simulink model "main_simulink"  (R2022a)
settings: Solver=VariableStepAuto  StartTime=0.0  StopTime=8  RelTol=1e-3
values from neighbouring files (symbols this model uses):
  A = 24    [main.m]
  a = 18    [main.m]
  b = 8    [main.m]
libraries: slpidlib x2, simulink_extras x2
settings Model: Creator=240818  LastModifiedBy=punk
settings DebuggingCC: UnconnectedInputMsg=warning  UnconnectedOutputMsg=warning  UnconnectedLineMsg=warning
settings RTWCC: DLArmComputeVersion=19.05

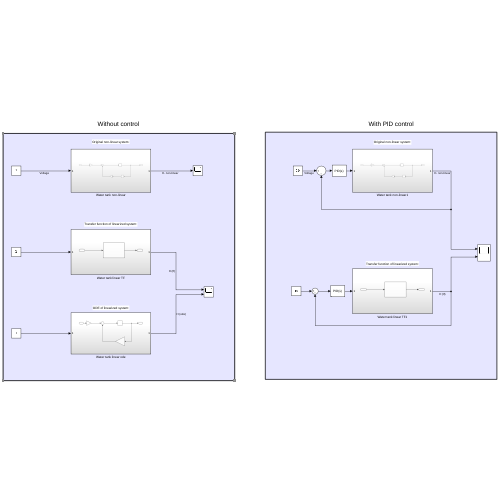
[thumbnail: Simulink's stored preview of the top-level diagram]
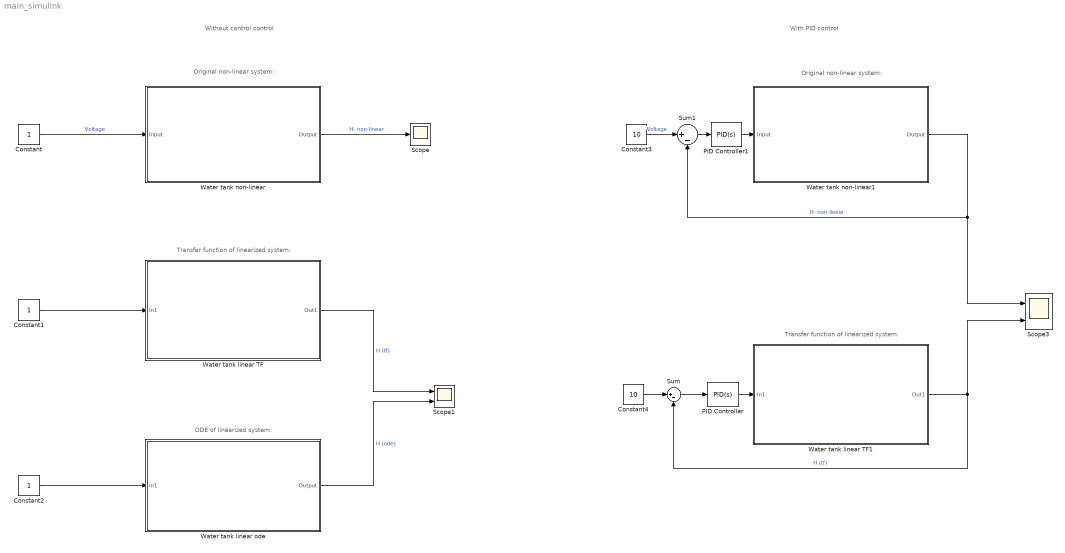
== system main_simulink ==
  note: With PID control
  note: ODE of linearized system:
  note: Transfer function of linearized system:
  note: Original non-linear system:
  note: Transfer function of linearized system:
  note: Original non-linear system:
  note: Without control control
  Constant : Constant
  Constant1 : Constant
  Constant2 : Constant
  Constant3 : Constant  Value=10
  Constant4 : Constant  Value=10
  PID Controller : slpidlib/PID Controller  Controller=PID  Form=Parallel  TimeDomain=Continuous-time  UseExternalTs=off  SampleTime=-1  IntegratorMethod=Forward Euler  FilterMethod=Forward Euler  ControllerParametersSource=internal  P=15  I=5  UseKiTs=off  D=1  N=0  UseFilter=on  TunerSelectOption=Transfer Function Based (PID Tuner App)  InitialConditionSource=internal  InitialConditionForIntegrator=0  InitialConditionForFilter=0  DifferentiatorICPrevScaledInput=0  ExternalReset=none  TrackingMode=off  Kt=1  LimitOutput=off  SatLimitsSource=internal  UpperSaturationLimit=inf  LowerSaturationLimit=-inf  LinearizeAsGain=on  AntiWindupMode=none  Kb=1  POutMin=[]  POutMax=[]  IOutMin=[]  IOutMax=[]  DOutMin=[]  DOutMax=[]  NOutMin=[]  NOutMax=[]  SumOutMin=[]  SumOutMax=[]  SaturationOutMin=[]  SaturationOutMax=[]  PParamMin=[]  PParamMax=[]  IParamMin=[]  IParamMax=[]  DParamMin=[]  DParamMax=[]  NParamMin=[]  NParamMax=[]  KbParamMin=[]  KbParamMax=[]  KtParamMin=[]  KtParamMax=[]  KbOutMin=[]  KbOutMax=[]  KtOutMin=[]  KtOutMax=[]  IntegratorOutMin=[]  IntegratorOutMax=[]  FilterOutMin=[]  FilterOutMax=[]  SumI1OutMin=[]  SumI1OutMax=[]  SumI2OutMin=[]  SumI2OutMax=[]  SumI3OutMin=[]  SumI3OutMax=[]  SumI4OutMin=[]  SumI4OutMax=[]  SumDOutMin=[]  SumDOutMax=[]  DifferentiatorOutMin=[]  DifferentiatorOutMax=[]  FilterDiffOutCoefMin=[]  FilterDiffOutCoefMax=[]  ReciprocalOutMin=[]  ReciprocalOutMax=[]  SumDenOutMin=[]  SumDenOutMax=[]  SumNumOutMin=[]  SumNumOutMax=[]  DivideOutMin=[]  DivideOutMax=[]  UdiffTsProdOutMin=[]  UdiffTsProdOutMax=[]  NTsProdOutMin=[]  NTsProdOutMax=[]  UintegralTsProdOutMin=[]  UintegralTsProdOutMax=[]  UngainTsProdOutMin=[]  UngainTsProdOutMax=[]  ClampingZeroOutDataTypeStr=Inherit: Inherit via back propagation  ClampingZeroOutMin=[]  ClampingZeroOutMax=[]  FilterDenConstantOutDataTypeStr=Inherit: Inherit via back propagation  FilterDenConstantOutMin=[]  FilterDenConstantOutMax=[]  PCopyOutDataTypeStr=Inherit: Inherit via back propagation  PCopyOutMin=[]  PCopyOutMax=[]  NCopyOutDataTypeStr=Inherit: Inherit via back propagation  NCopyOutMin=[]  NCopyOutMax=[]  IntegratorContinuousStateAttributes=''  IntegratorStateMustResolveToSignalObject=off  IntegratorRTWStateStorageClass=Auto  FilterContinuousStateAttributes=''  FilterStateMustResolveToSignalObject=off  FilterRTWStateStorageClass=Auto  ParallelPVariant=InternalParameters  IdealPVariant=Disabled  IVariant=InternalParameters  DVariant=InternalParameters  IntegratorVariant=Continuous  SatVariant=Disabled  AWVariant=Passthrough  PCopyVariant=Disabled  TRVariant=Disabled  FdbkBlocksVariant=Forward  IdealPFdbkVariant=Disabled  SatFdbkVariant=Disabled  DerivativeFilterVariant=ContFilter  NVariant=InternalParameters  NCopyVariant=Disabled  FilterICVariant=InternalICsFilter  IntegratorICVariant=InternalICs  ExternalResetVariant=Disabled  TRSumVariant=Passthrough  SumFdbkVariant=Disabled  SumVariant=Sum_PID  TsampFilterVariant=InternalTs  TsampNgainVariant=Passthrough  TsampIntegralVariant=Passthrough  ExternalSaturationOutDataTypeStr=Inherit: Same as second input  aMode=0
  PID Controller1 : slpidlib/PID Controller  Controller=PID  Form=Parallel  TimeDomain=Continuous-time  UseExternalTs=off  SampleTime=-1  IntegratorMethod=Forward Euler  FilterMethod=Forward Euler  ControllerParametersSource=internal  P=15  I=5  UseKiTs=off  D=1  N=0  UseFilter=on  TunerSelectOption=Transfer Function Based (PID Tuner App)  InitialConditionSource=internal  InitialConditionForIntegrator=0  InitialConditionForFilter=0  DifferentiatorICPrevScaledInput=0  ExternalReset=none  TrackingMode=off  Kt=1  LimitOutput=off  SatLimitsSource=internal  UpperSaturationLimit=inf  LowerSaturationLimit=-inf  LinearizeAsGain=on  AntiWindupMode=none  Kb=1  POutMin=[]  POutMax=[]  IOutMin=[]  IOutMax=[]  DOutMin=[]  DOutMax=[]  NOutMin=[]  NOutMax=[]  SumOutMin=[]  SumOutMax=[]  SaturationOutMin=[]  SaturationOutMax=[]  PParamMin=[]  PParamMax=[]  IParamMin=[]  IParamMax=[]  DParamMin=[]  DParamMax=[]  NParamMin=[]  NParamMax=[]  KbParamMin=[]  KbParamMax=[]  KtParamMin=[]  KtParamMax=[]  KbOutMin=[]  KbOutMax=[]  KtOutMin=[]  KtOutMax=[]  IntegratorOutMin=[]  IntegratorOutMax=[]  FilterOutMin=[]  FilterOutMax=[]  SumI1OutMin=[]  SumI1OutMax=[]  SumI2OutMin=[]  SumI2OutMax=[]  SumI3OutMin=[]  SumI3OutMax=[]  SumI4OutMin=[]  SumI4OutMax=[]  SumDOutMin=[]  SumDOutMax=[]  DifferentiatorOutMin=[]  DifferentiatorOutMax=[]  FilterDiffOutCoefMin=[]  FilterDiffOutCoefMax=[]  ReciprocalOutMin=[]  ReciprocalOutMax=[]  SumDenOutMin=[]  SumDenOutMax=[]  SumNumOutMin=[]  SumNumOutMax=[]  DivideOutMin=[]  DivideOutMax=[]  UdiffTsProdOutMin=[]  UdiffTsProdOutMax=[]  NTsProdOutMin=[]  NTsProdOutMax=[]  UintegralTsProdOutMin=[]  UintegralTsProdOutMax=[]  UngainTsProdOutMin=[]  UngainTsProdOutMax=[]  ClampingZeroOutDataTypeStr=Inherit: Inherit via back propagation  ClampingZeroOutMin=[]  ClampingZeroOutMax=[]  FilterDenConstantOutDataTypeStr=Inherit: Inherit via back propagation  FilterDenConstantOutMin=[]  FilterDenConstantOutMax=[]  PCopyOutDataTypeStr=Inherit: Inherit via back propagation  PCopyOutMin=[]  PCopyOutMax=[]  NCopyOutDataTypeStr=Inherit: Inherit via back propagation  NCopyOutMin=[]  NCopyOutMax=[]  IntegratorContinuousStateAttributes=''  IntegratorStateMustResolveToSignalObject=off  IntegratorRTWStateStorageClass=Auto  FilterContinuousStateAttributes=''  FilterStateMustResolveToSignalObject=off  FilterRTWStateStorageClass=Auto  ParallelPVariant=InternalParameters  IdealPVariant=Disabled  IVariant=InternalParameters  DVariant=InternalParameters  IntegratorVariant=Continuous  SatVariant=Disabled  AWVariant=Passthrough  PCopyVariant=Disabled  TRVariant=Disabled  FdbkBlocksVariant=Forward  IdealPFdbkVariant=Disabled  SatFdbkVariant=Disabled  DerivativeFilterVariant=ContFilter  NVariant=InternalParameters  NCopyVariant=Disabled  FilterICVariant=InternalICsFilter  IntegratorICVariant=InternalICs  ExternalResetVariant=Disabled  TRSumVariant=Passthrough  SumFdbkVariant=Disabled  SumVariant=Sum_PID  TsampFilterVariant=InternalTs  TsampNgainVariant=Passthrough  TsampIntegralVariant=Passthrough  ExternalSaturationOutDataTypeStr=Inherit: Same as second input  aMode=0
  Scope : Scope
  Scope1 : Scope  NumInputPorts=2
  Scope3 : Scope  NumInputPorts=2
  Sum : Sum  Inputs=|+-
  Sum1 : Sum  Inputs=|+-
  Water tank linear TF : Subsystem
  Water tank linear TF1 : Subsystem
  Water tank linear ode : Subsystem
  Water tank non-linear : Subsystem
  Water tank non-linear1 : Subsystem
  wires:
  Constant/1 -> Water tank non-linear/1(Input)  "Voltage"
  Water tank non-linear/1(Output) -> Scope/1  "H- non-linear"
  Constant1/1 -> Water tank linear TF/1(In1)
  Water tank linear TF/1(Out1) -> Scope1/1  "H (tf)"
  Constant2/1 -> Water tank linear ode/1(In1)
  Water tank linear ode/1(Output) -> Scope1/2  "H (ode)"
  Constant3/1 -> Sum1/1  "Voltage"
  Water tank linear TF1/1(Out1) -> Sum/2, Scope3/2  "H (tf)"
  PID Controller/1 -> Water tank linear TF1/1(In1)
  Sum/1 -> PID Controller/1
  Constant4/1 -> Sum/1
  PID Controller1/1 -> Water tank non-linear1/1(Input)
  Sum1/1 -> PID Controller1/1
  Water tank non-linear1/1(Output) -> Scope3/1, Sum1/2  "H- non-linear"

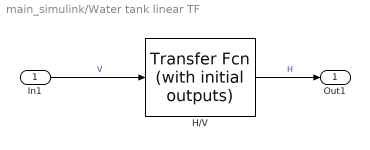
== system main_simulink/Water tank linear TF ==
  In1 : Inport
  H/V : simulink_extras/Additional Linear/Transfer Fcn (with initial outputs)  N=[b/A]  D="[1  0.16*(a/A)]"  Y0=10  U0=0
  Out1 : Outport
  wires:
  In1/1 -> H/V/1  "V"
  H/V/1 -> Out1/1  "H"

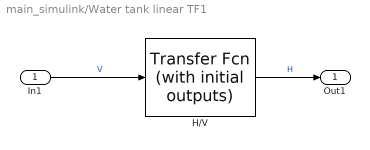
== system main_simulink/Water tank linear TF1 ==
  In1 : Inport
  H/V : simulink_extras/Additional Linear/Transfer Fcn (with initial outputs)  N=[b/A]  D="[1  1/(2*sqrt(10))*(a/A)]"  Y0=9  U0=0
  Out1 : Outport
  wires:
  In1/1 -> H/V/1  "V"
  H/V/1 -> Out1/1  "H"

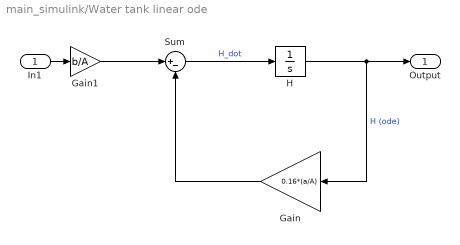
== system main_simulink/Water tank linear ode ==
  In1 : Inport
  Gain : Gain  Gain=0.16*(a/A)
  Gain1 : Gain  Gain=b/A
  H : Integrator  InitialCondition=10
  Sum : Sum  Inputs=|+-
  Output : Outport
  wires:
  H/1 -> Output/1, Gain/1  "H (ode)"
  In1/1 -> Gain1/1
  Gain/1 -> Sum/2
  Sum/1 -> H/1  "H_dot"
  Gain1/1 -> Sum/1

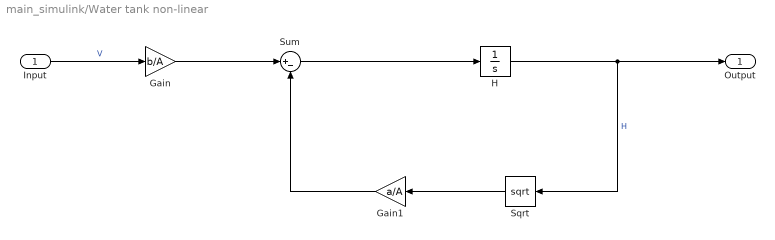
== system main_simulink/Water tank non-linear ==
  Input : Inport
  Gain : Gain  Gain=b/A
  Gain1 : Gain  Gain=a/A
  H : Integrator  InitialCondition=10
  Sqrt : Sqrt
  Sum : Sum  Inputs=|+-
  Output : Outport
  wires:
  Gain1/1 -> Sum/2
  H/1 -> Sqrt/1, Output/1  "H"
  Sum/1 -> H/1
  Sqrt/1 -> Gain1/1
  Input/1 -> Gain/1  "V"
  Gain/1 -> Sum/1

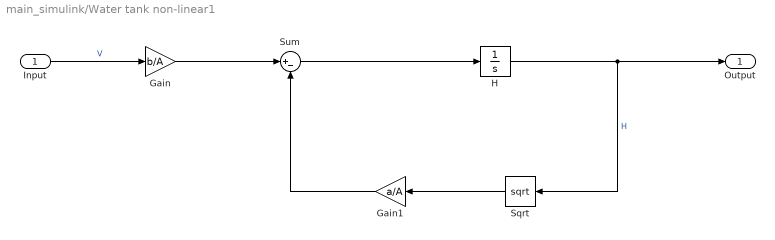
== system main_simulink/Water tank non-linear1 ==
  Input : Inport
  Gain : Gain  Gain=b/A
  Gain1 : Gain  Gain=a/A
  H : Integrator  InitialCondition=9
  Sqrt : Sqrt
  Sum : Sum  Inputs=|+-
  Output : Outport
  wires:
  Gain1/1 -> Sum/2
  H/1 -> Sqrt/1, Output/1  "H"
  Sum/1 -> H/1
  Sqrt/1 -> Gain1/1
  Input/1 -> Gain/1  "V"
  Gain/1 -> Sum/1
